simulink model "sysID"  (R2018b)
settings: Solver=VariableStepAuto  StartTime=0.0  StopTime=10000  RelTol=1e-3
libraries: cstblocks x1
settings Model: Creator=lenovo  LastModifiedBy=lenovo
settings OptimizationCC: DefaultParameterBehavior=Inlined  BufferReuse=off
settings DebuggingCC: InitInArrayFormatMsg=none

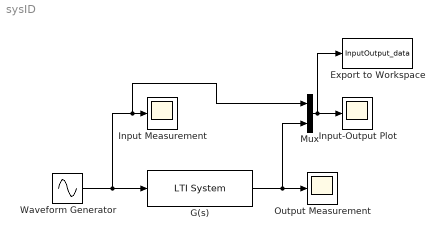
== system sysID ==
  Export to Workspace : ToWorkspace  VariableName=InputOutput_data  SaveFormat=Timeseries  SampleTime=-1
  G(s) : cstblocks/LTI System  sys=G1_pade  IC=[]
  Input Measurement : Scope
  Input-Output Plot : Scope
  Mux : Mux  Inputs=2
  Output Measurement : Scope
  Waveform Generator : Sin  Frequency=8e-04  SampleTime=0
  wires:
  G(s)/1 -> Mux/2, Output Measurement/1
  Waveform Generator/1 -> Mux/1, Input Measurement/1, G(s)/1
  Mux/1 -> Export to Workspace/1, Input-Output Plot/1
